simulink model "INIT"  (R2014a)
settings: Solver=ode45  StartTime=0.0  StopTime=10.0  RelTol=1e-3
undefined symbols (not defined in the file): dt, dtheta1_throw_traj, Kd1, Kp1, theta1_init_traj, theta1_throw_traj, Ts_trah_throw, Ts_traj
libraries: legonxtlib x2, simulink_extras x1, cstblocks x1
settings Model: SimulationMode=external  Creator=yutongfeng  LastModifiedBy=yutongfeng

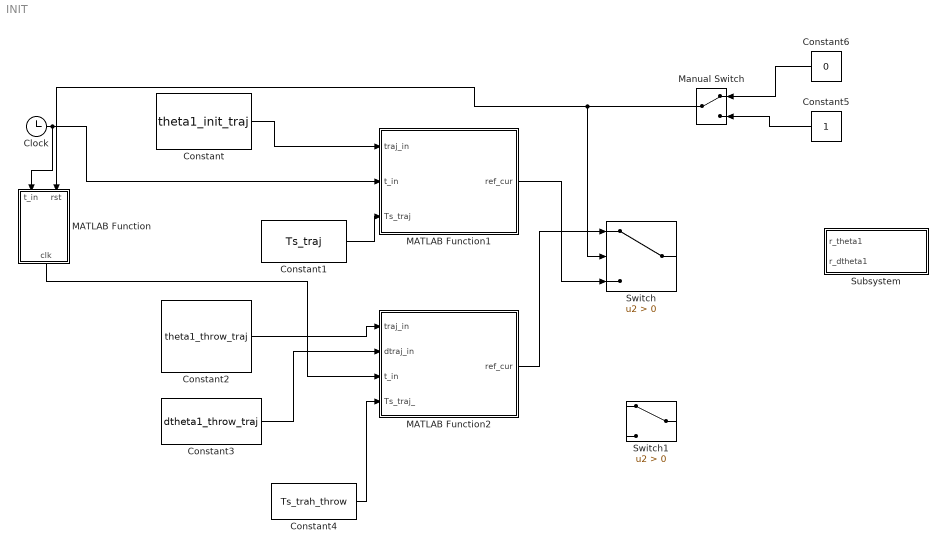
== system INIT ==
  Clock : Clock
  Constant : Constant  Value=theta1_init_traj  SampleTime=dt
  Constant1 : Constant  Value=Ts_traj  SampleTime=dt
  Constant2 : Constant  Value=theta1_throw_traj  SampleTime=dt
  Constant3 : Constant  Value=dtheta1_throw_traj  SampleTime=dt
  Constant4 : Constant  Value=Ts_trah_throw  SampleTime=dt
  Constant5 : Constant  SampleTime=dt
  Constant6 : Constant  Value=0  SampleTime=dt
  MATLAB Function : MATLAB Function  TreatAsAtomicUnit=on
  MATLAB Function1 : MATLAB Function  TreatAsAtomicUnit=on
  MATLAB Function2 : MATLAB Function  TreatAsAtomicUnit=on
  Manual Switch : ManualSwitch
  Subsystem : Subsystem
  Switch : Switch  Criteria=u2 > Threshold
  Switch1 : Switch  Criteria=u2 > Threshold
  wires:
  Constant/1 -> MATLAB Function1/1(traj_in)
  Clock/1 -> MATLAB Function/1(t_in), MATLAB Function1/2(t_in)
  Constant1/1 -> MATLAB Function1/3(Ts_traj)
  Constant2/1 -> MATLAB Function2/1(traj_in)
  Constant3/1 -> MATLAB Function2/2(dtraj_in)
  MATLAB Function/1(clk) -> MATLAB Function2/3(t_in)
  Constant4/1 -> MATLAB Function2/4(Ts_traj_)
  MATLAB Function1/1(ref_cur) -> Switch/3
  MATLAB Function2/1(ref_cur) -> Switch/1
  Manual Switch/1 -> Switch/2, MATLAB Function/2(rst)
  Constant6/1 -> Manual Switch/1
  Constant5/1 -> Manual Switch/2

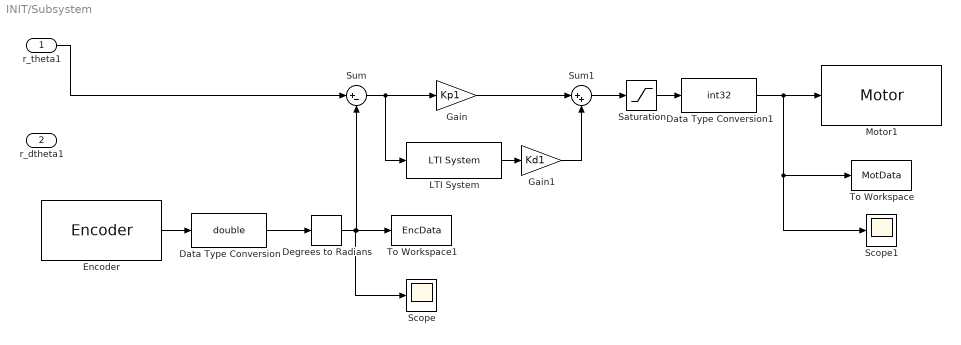
== system INIT/Subsystem ==
  r_theta1 : Inport
  r_dtheta1 : Inport  Port=2
  Data Type Conversion : DataTypeConversion  OutMin=-100  OutMax=100  OutDataTypeStr=double
  Data Type Conversion1 : DataTypeConversion  OutMin=-100  OutMax=100  OutDataTypeStr=int32
  Degrees to Radians : simulink_extras/Transformations/Degrees to Radians
  Encoder : legonxtlib/Encoder  portNumber=B  opMode=No reset  sampleTime=dt
  Gain : Gain  Gain=Kp1
  Gain1 : Gain  Gain=Kd1
  LTI System : cstblocks/LTI System  sys=dttf  IC=[]
  Motor1 : legonxtlib/Motor  sportNumber=B  sstopAction=Brake
  Saturation : Saturate  UpperLimit=100  LowerLimit=-100  SampleTime=dt
  Scope : Scope
      settings: YMin=-0.5  YMax=6.5
  Scope1 : Scope
      settings: YMin=2.85  YMax=3.15
  Sum : Sum  Inputs=|+-
  Sum1 : Sum  Inputs=|++
  To Workspace : ToWorkspace  VariableName=MotData  SaveFormat=Structure With Time  SampleTime=dt
  To Workspace1 : ToWorkspace  VariableName=EncData  SaveFormat=Structure With Time  SampleTime=dt
  wires:
  Saturation/1 -> Data Type Conversion1/1
  Data Type Conversion/1 -> Degrees to Radians/1
  Degrees to Radians/1 -> To Workspace1/1, Sum/2, Scope/1
  Data Type Conversion1/1 -> Scope1/1, To Workspace/1, Motor1/1
  Encoder/1 -> Data Type Conversion/1
  Sum/1 -> Gain/1, LTI System/1
  Gain/1 -> Sum1/1
  Sum1/1 -> Saturation/1
  r_theta1/1 -> Sum/1
  LTI System/1 -> Gain1/1
  Gain1/1 -> Sum1/2

== matlab function INIT/MATLAB Function1 ==
  data: traj_in input; ref_cur output; t_in input; Ts_traj input
function ref_cur = fcn(traj_in, t_in,Ts_traj)
%#codegen

ref_cur= u;

== matlab function INIT/MATLAB Function ==
  data: t_in input; clk output; rst input
function clk = fcn(t_in, rst)
persistent t_off last_rst
if isempty(t_off)
 t_off = 0;
end
if isempty(last_rst)
 last_rst = 0;
end
%if rest switch was pressed, use current time as t_offset
if abs(rst - last_rst) ~= 0
 t_off = t_in;
end
clk = t_in - t_off; %output clock
last_rst = rst; %update reset var

== matlab function INIT/MATLAB Function2 ==
  data: traj_in input; dtraj_in input; ref_cur output; t_in input; Ts_traj_ input
function ref_cur = fcn(traj_in,dtraj_in, t_in,Ts_traj_)
%#codegen

ref_cur= u;
